simulink model "Room_thermal_ML_control"  (R2021a)
settings: Solver=ode1  StartTime=0.0  StopTime=259200  FixedStep=60  RelTol=1e-3
libraries: simulink x1
settings Model: Creator=OGHOSA  LastModifiedBy=OGHOSA

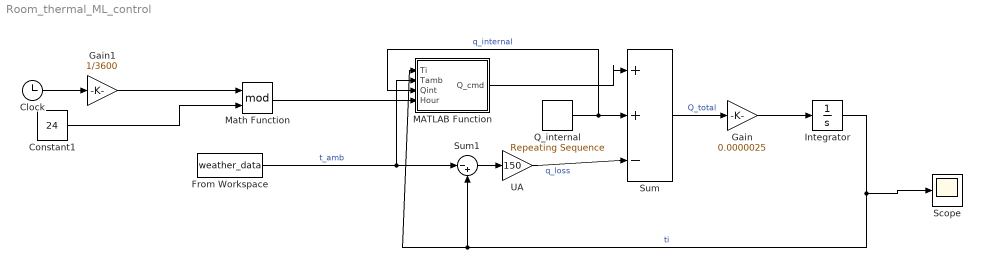
== system Room_thermal_ML_control ==
  Clock : Clock
  Constant1 : Constant  Value=24
  From Workspace : FromWorkspace  VariableName=weather_data
  Gain : Gain  Gain=0.0000025
  Gain1 : Gain  Gain=1/3600
  Integrator : Integrator  InitialCondition=293.15
  MATLAB Function : MATLAB Function  TreatAsAtomicUnit=on
  Math Function : Math  Operator=mod  SaturateOnIntegerOverflow=on
  Q_internal : simulink/Sources/Repeating Sequence  rep_seq_t=[0, 28000, 64000, 86400]  rep_seq_y=[100, 500, 100, 100]
  Scope : Scope
  Sum : Sum  Inputs=+|+|-
  Sum1 : Sum  Inputs=|-+
  UA : Gain  Gain=150
  wires:
  Sum/1 -> Gain/1  "Q_total"
  Gain/1 -> Integrator/1
  Q_internal/1 -> MATLAB Function/3(Qint), Sum/2  "q_internal"
  Integrator/1 -> Scope/1, MATLAB Function/1(Ti), Sum1/2  "ti"
  Sum1/1 -> UA/1
  UA/1 -> Sum/3  "q_loss"
  From Workspace/1 -> Sum1/1, MATLAB Function/2(Tamb)  "t_amb"
  Math Function/1 -> MATLAB Function/4(Hour)
  Gain1/1 -> Math Function/1
  Clock/1 -> Gain1/1
  Constant1/1 -> Math Function/2
  MATLAB Function/1(Q_cmd) -> Sum/1

== matlab function Room_thermal_ML_control/MATLAB Function ==
  data: Ti input; Q_cmd output; Tamb input; Qint input; Hour input
function Q_cmd = fcn(Ti, Tamb, Qint, Hour)
    coder.extrinsic('py.thermal_api.predict_next_temp');

    Q_max = 3000;
    Q_off = 0;
    T_set = 295.15;
    
    % --- SAFETY BAND (Hybrid Control) ---
    % If we are very cold (more than 2 degrees below setpoint), FORCE HEAT.
    % This overcomes the "short horizon" issue and ensures we reach the operating zone.
    if Ti < (T_set - 2.0)
        Q_cmd = Q_max;
        return; % Exit early
    end
    
    % --- ML PRECISION CONTROL ---
    % We only use ML when we are close to the target to prevent overshoot
    % and optimize energy.
    
    pred_off = 0.0;
    pred_on = 0.0;
    
    % Scenario A: Predict OFF
    pred_off = py.thermal_api.predict_next_temp(Ti, Q_off, Tamb, Qint, Hour);
    T_next_OFF = double(pred_off); 
    
    % Scenario B: Predict ON
    pred_on = py.thermal_api.predict_next_temp(Ti, Q_max, Tamb, Qint, Hour);
    T_next_ON = double(pred_on);
    
    % Optimization
    Error_OFF = abs(T_next_OFF - T_set);
    Error_ON  = abs(T_next_ON - T_set);
    
    if Error_ON < Error_OFF
        Q_cmd = Q_max;
    else
        Q_cmd = Q_off;
    end
end
